simulink subsystem "NoSteering"  (R2022b)
settings: Solver=VariableStepAuto  StartTime=0.0  StopTime=10.0  RelTol=1e-3
settings Model: ModifiedByFormat=The MathWorks, Inc.  Creator=The MathWorks, Inc.  LastModifiedBy=The MathWorks, Inc.

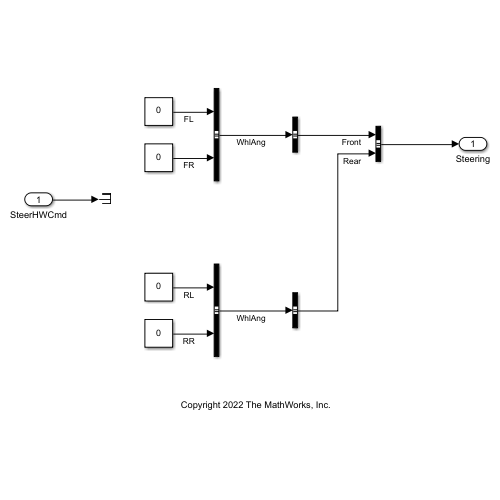
[thumbnail: Simulink's stored preview of the top-level diagram]
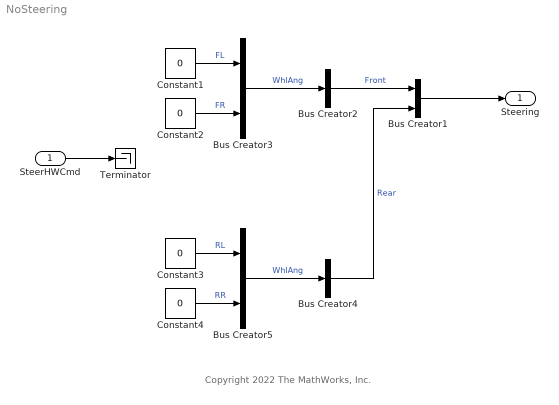
== system NoSteering ==
  note: Copyright 2022 The MathWorks, Inc.
  SteerHWCmd : Inport
  Bus Creator1 : BusCreator  Inputs=2
  Bus Creator2 : BusCreator  Inputs=1
  Bus Creator3 : BusCreator  Inputs=2
  Bus Creator4 : BusCreator  Inputs=1
  Bus Creator5 : BusCreator  Inputs=2
  Constant{1..4} (4 alike) : Constant  Value=0  SampleTime=-1
  Terminator : Terminator
  Steering : Outport
  wires:
  Bus Creator3/1 -> Bus Creator2/1  "WhlAng"
  Bus Creator2/1 -> Bus Creator1/1  "Front"
  Bus Creator4/1 -> Bus Creator1/2  "Rear"
  Constant4/1 -> Bus Creator5/2  "RR"
  Bus Creator5/1 -> Bus Creator4/1  "WhlAng"
  Constant2/1 -> Bus Creator3/2  "FR"
  Constant1/1 -> Bus Creator3/1  "FL"
  Constant3/1 -> Bus Creator5/1  "RL"
  Bus Creator1/1 -> Steering/1
  SteerHWCmd/1 -> Terminator/1
